simulink library "STRUCT_MDL"  (R2015a)
settings: Solver=ode45  StartTime=0.0  StopTime=10.0  RelTol=1e-3
libraries: AF_MDL x2, FIN_MDL x1, NC_MDL x1
settings Model: Creator=Andrew  LastModifiedBy=Andrew

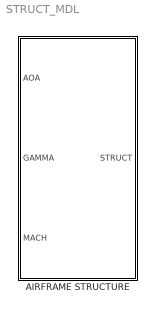
== system STRUCT_MDL ==
  AIRFRAME STRUCTURE : Subsystem

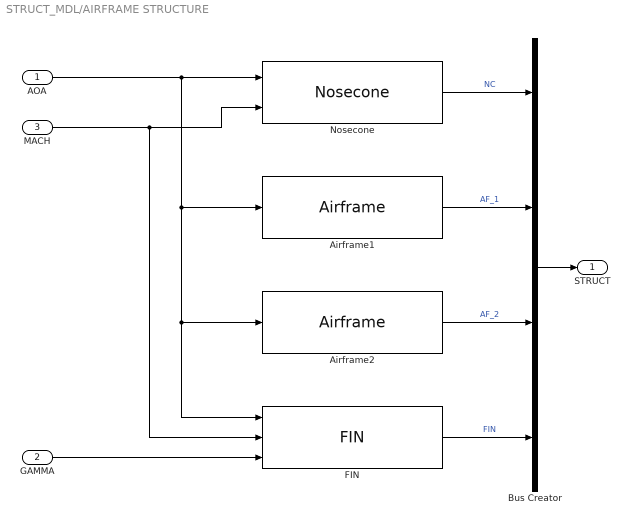
== system STRUCT_MDL/AIRFRAME STRUCTURE ==
  AOA : Inport
  GAMMA : Inport  Port=2
  MACH : Inport  Port=3
  Airframe1 : AF_MDL/Airframe  AF=AF_1
  Airframe2 : AF_MDL/Airframe  AF=AF_2
  Bus Creator : BusCreator
  FIN : FIN_MDL/FIN  FIN=FIN
  Nosecone : NC_MDL/Nosecone  NC=NC
  STRUCT : Outport
  wires:
  Airframe2/1 -> Bus Creator/3  "AF_2"
  Nosecone/1 -> Bus Creator/1  "NC"
  MACH/1 -> Nosecone/2, FIN/2
  AOA/1 -> Nosecone/1, Airframe1/1, Airframe2/1, FIN/1
  Bus Creator/1 -> STRUCT/1
  GAMMA/1 -> FIN/3
  FIN/1 -> Bus Creator/4  "FIN"
  Airframe1/1 -> Bus Creator/2  "AF_1"
